simulink model "simulink_s2_export_2020a"  (R2020a)
settings: Solver=VariableStepAuto  StartTime=0.0  StopTime=10.0  RelTol=1e-3
undefined symbols (not defined in the file): A0, K, perturbation_step_amplitude, T, u0, y0
settings Model: Creator=Admin  LastModifiedBy=ajj
settings DebuggingCC: UnconnectedInputMsg=none  UnconnectedOutputMsg=none  UnconnectedLineMsg=none
settings ModelReferenceCC: EnableRefExpFcnMdlSchedulingChecks=off
settings RTWCC: Description=Generic Real-Time Target

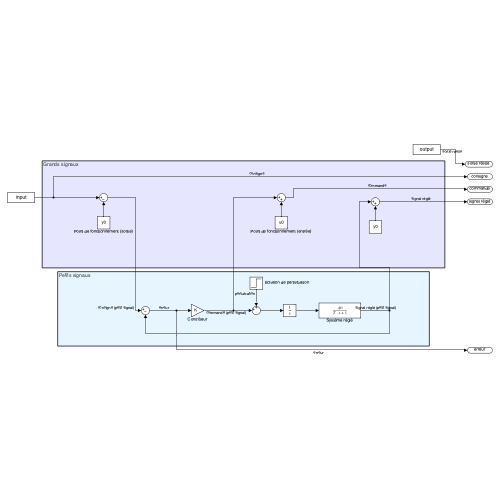
[thumbnail: Simulink's stored preview of the top-level diagram]
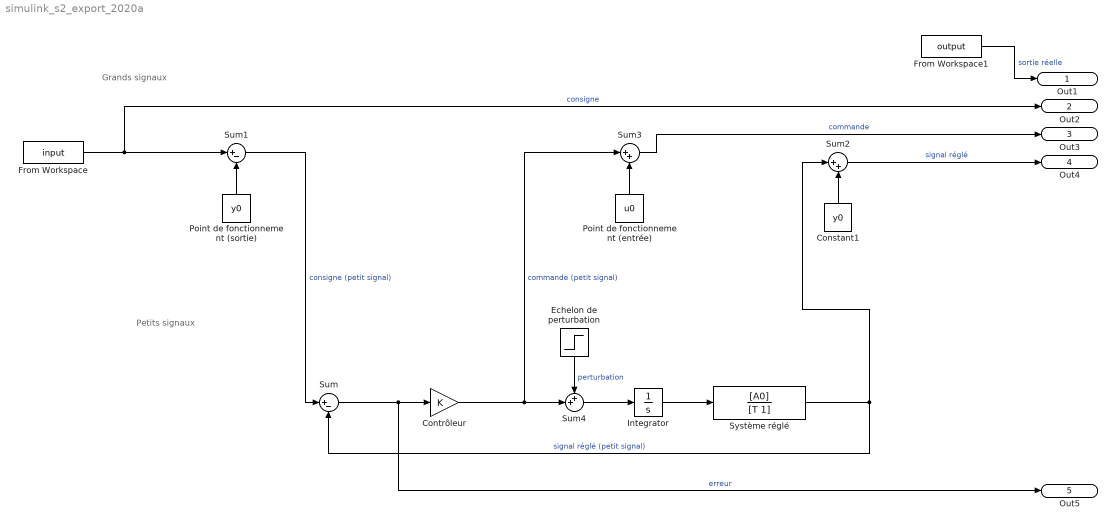
== system simulink_s2_export_2020a ==
  note: Petits signaux
  note: Grands signaux
  Constant1 : Constant  Value=y0
  Contrôleur : Gain  Gain=K
  Echelon de perturbation : Step  After=perturbation_step_amplitude  SampleTime=0
  From Workspace : FromWorkspace  VariableName=input
  From Workspace1 : FromWorkspace  VariableName=output
  Integrator : Integrator
  Point de fonctionnement (entrée) : Constant  Value=u0
  Point de fonctionnement (sortie) : Constant  Value=y0
  Sum : Sum  Inputs=|+-
  Sum1 : Sum  Inputs=|+-
  Sum2 : Sum  Inputs=|++
  Sum3 : Sum  Inputs=|++
  Sum4 : Sum  Inputs=++|
  Système réglé : TransferFcn  Numerator=[A0]  Denominator=[T 1]
  Out1 : Outport
  Out2 : Outport  Port=2
  Out3 : Outport  Port=3
  Out4 : Outport  Port=4
  Out5 : Outport  Port=5
  wires:
  Sum/1 -> Out5/1, Contrôleur/1  "erreur"
  Contrôleur/1 -> Sum4/2, Sum3/1  "commande (petit signal)"
  Système réglé/1 -> Sum2/1, Sum/2  "signal réglé (petit signal)"
  Constant1/1 -> Sum2/2
  Sum2/1 -> Out4/1  "signal réglé"
  From Workspace/1 -> Sum1/1, Out2/1  "consigne"
  Sum1/1 -> Sum/1  "consigne (petit signal)"
  Point de fonctionnement (sortie)/1 -> Sum1/2
  Point de fonctionnement (entrée)/1 -> Sum3/2
  Sum3/1 -> Out3/1  "commande"
  Sum4/1 -> Integrator/1
  Integrator/1 -> Système réglé/1
  Echelon de perturbation/1 -> Sum4/1  "perturbation"
  From Workspace1/1 -> Out1/1  "sortie réelle"
